simulink model "lanechange"  (R2021a)
settings: Solver=ode45  StartTime=0.0  StopTime=10.0  RelTol=1e-3  EnableMultiTasking=on
libraries: simulink x2
settings Model: Creator=pic  LastModifiedBy=User
settings SolverCC: AlgebraicLoopSolver=TrustRegion
settings DataIOCC: LimitDataPoints=on  SaveFormat=Array  SignalLoggingSaveFormat=ModelDataLogs  SignalLogging=off  DSMLogging=off  VisualizeSimOutput=off  TimeSaveName=t  OutputSaveName=y
settings OptimizationCC: ExpressionDepthLimit=2147483647  LifeSpan=inf
settings DebuggingCC: UnderspecifiedInitializationDetection=Classic  MergeDetectMultiDrivingBlocksExec=none  SolverPrmCheckMsg=warning  FcnCallInpInsideContextMsg=warning  AllowSymbolicDim=off  StateNameClashWarn=warning  SFUnexpectedBacktrackingDiag=warning  SFNoUnconditionalDefaultTransitionDiag=warning  SFMachineParentedDataDiag=warning  ArithmeticOperatorsInVariantConditions=warning
settings HardwareCC: ProdBitPerPointer=32  ProdBitPerSizeT=32  ProdBitPerPtrDiffT=32  ProdLargestAtomicFloat=None  ProdIntDivRoundTo=Undefined  ProdEndianess=Unspecified  ProdWordSize=32  ProdHWDeviceType=32-bit Generic
settings ModelReferenceCC: PropagateSignalLabelsOutOfModel=off
settings SFSimCC: SimUseLocalCustomCode=off  CustomCodeUndefinedFunction=UseInterfaceOnly
settings RTWCC: RTWUseLocalCustomCode=off
settings CodeAppCC: StateflowObjectComments=on
settings GRTTargetCC: TargetLangStandard=C89/C90 (ANSI)  CombineOutputUpdateFcns=off  GRTInterface=on
settings ConfigComp: CovMetricSettings=dw  CovSaveCumulativeToWorkspaceVar=on  CovSaveSingleToWorkspaceVar=on  CovExternalEMLEnable=off

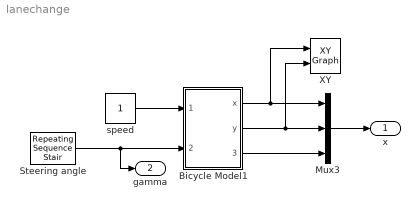
== system lanechange ==
  Bicycle Model1 : Subsystem
  Mux3 : Mux  Inputs=3
  Steering angle : simulink/Sources/Repeating Sequence Stair  OutValues=[0 0 0 0.5 0 -0.5 0 0 0 0]  tsamp=1  OutMin=[]  OutMax=[]  OutDataTypeStr=double  OutputDataTypeScalingMode=Specify via dialog  OutDataType=double  ConRadixGroup=Best Precision: Vector-wise  OutScaling=2^-12
  XY : simulink/Sinks/XY Graph  xmin=0  xmax=10  ymin=0  ymax=4  st=-1
  speed : Constant  VectorParams1D=off  SampleTime=0.02
  x : Outport
  gamma : Outport  Port=2
  wires:
  Steering angle/1 -> Bicycle Model1/2(gamma), gamma/1
  speed/1 -> Bicycle Model1/1(velocity)
  Bicycle Model1/3(theta) -> Mux3/3
  Bicycle Model1/1(x) -> Mux3/1, XY/1
  Bicycle Model1/2(y) -> Mux3/2, XY/2
  Mux3/1 -> x/1

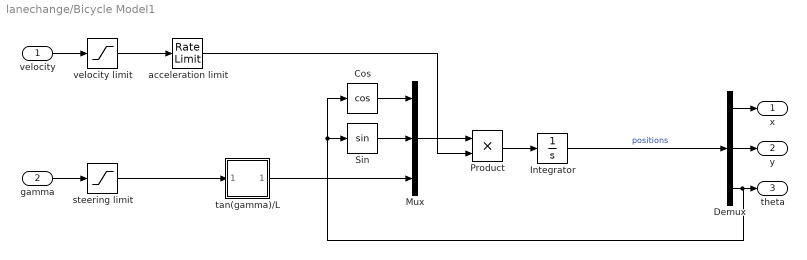
== system lanechange/Bicycle Model1 ==
  velocity : Inport
  gamma : Inport  Port=2
  Cos : Trigonometry  Operator=cos
  Demux : Demux  Outputs=3
  Integrator : Integrator  InitialCondition=[0 0 0]
  Mux : Mux  Inputs=3
  Product : Product
  Sin : Trigonometry
  acceleration limit : RateLimiter  RisingSlewLimit=2  FallingSlewLimit=-2  SampleTimeMode=inherited
  steering limit : Saturate  UpperLimit=1  LowerLimit=-1
  tan(gamma)/L : Subsystem
  velocity limit : Saturate  UpperLimit=5  LowerLimit=-5
  x : Outport
  y : Outport  Port=2
  theta : Outport  Port=3
  wires:
  Sin/1 -> Mux/2
  Cos/1 -> Mux/1
  Demux/2 -> y/1
  Demux/1 -> x/1
  Demux/3 -> theta/1, Sin/1, Cos/1
  Integrator/1 -> Demux/1  "positions"
  Product/1 -> Integrator/1
  acceleration limit/1 -> Product/2
  Mux/1 -> Product/1
  tan(gamma)/L/1(Out1) -> Mux/3
  steering limit/1 -> tan(gamma)/L/1(In1)
  gamma/1 -> steering limit/1
  velocity limit/1 -> acceleration limit/1
  velocity/1 -> velocity limit/1

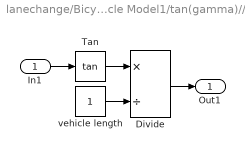
== system lanechange/Bicycle Model1/tan(gamma)//L ==
  In1 : Inport
  Divide : Product  Inputs=*/
  Tan : Trigonometry  Operator=tan
  vehicle length : Constant
  Out1 : Outport
  wires:
  Divide/1 -> Out1/1
  In1/1 -> Tan/1
  vehicle length/1 -> Divide/2
  Tan/1 -> Divide/1
